simulink model "lab1"  (R2024b)
settings: Solver=VariableStepAuto  StartTime=0.0  StopTime=20  RelTol=1e-3
libraries: dspswit3 x2
settings Model: Creator=Ahmad  LastModifiedBy=Ahmad

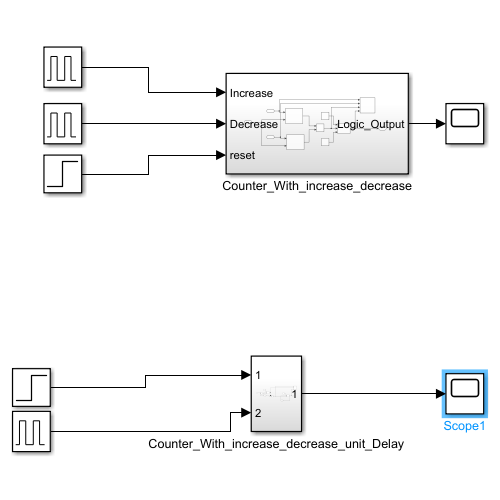
[thumbnail: Simulink's stored preview of the top-level diagram]
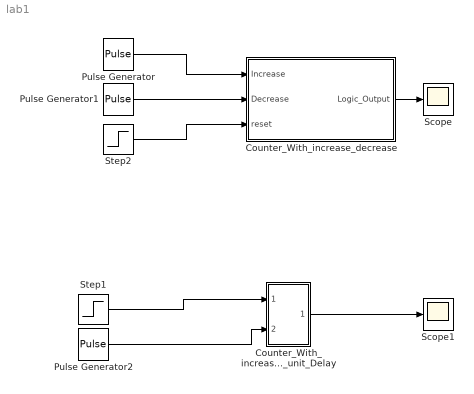
== system lab1 ==
  Counter_With_increase_decrease : Subsystem
  Counter_With_increase_decrease_unit_Delay : Subsystem
  Pulse Generator : DiscretePulseGenerator  PulseType=Time based  Period=1  PulseWidth=50
  Pulse Generator1 : DiscretePulseGenerator  PulseType=Time based  Period=6  PulseWidth=50
  Pulse Generator2 : DiscretePulseGenerator  PulseType=Time based  Period=6  PulseWidth=50
  Scope : Scope
  Scope1 : Scope
  Step1 : Step  SampleTime=1
  Step2 : Step  Time=8  SampleTime=0
  wires:
  Step1/1 -> Counter_With_increase_decrease_unit_Delay/1(In1)
  Pulse Generator/1 -> Counter_With_increase_decrease/1(Increase)
  Step2/1 -> Counter_With_increase_decrease/3(reset)
  Pulse Generator1/1 -> Counter_With_increase_decrease/2(Decrease)
  Counter_With_increase_decrease/1(Logic_Output) -> Scope/1
  Counter_With_increase_decrease_unit_Delay/1(Out1) -> Scope1/1
  Pulse Generator2/1 -> Counter_With_increase_decrease_unit_Delay/2(In2)

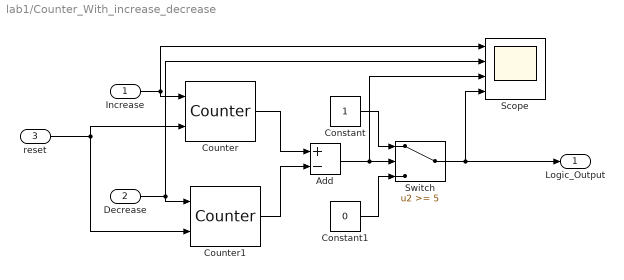
== system lab1/Counter_With_increase_decrease ==
  Increase : Inport
  Decrease : Inport  Port=2
  reset : Inport  Port=3
  Add : Sum  Inputs=+-
  Constant : Constant
  Constant1 : Constant  Value=0
  Counter : dspswit3/Counter  Direction=Up  CountEvent=Rising edge  CounterSize=User defined  MaxCount=255  InitialCount=0  Output=Count  HitValue=32  ResetInput=on  SamplesPerFrame=1  Ts=1  CntDtype=double  HitDtype=Logical
  Counter1 : dspswit3/Counter  Direction=Up  CountEvent=Rising edge  CounterSize=User defined  MaxCount=255  InitialCount=0  Output=Count  HitValue=32  ResetInput=on  SamplesPerFrame=1  Ts=1  CntDtype=double  HitDtype=Logical
  Scope : Scope  NumInputPorts=4
  Switch : Switch  Threshold=5  SaturateOnIntegerOverflow=off  InputSameDT=off
  Logic_Output : Outport
  wires:
  Decrease/1 -> Scope/2, Counter1/1
  Counter1/1 -> Add/2
  Add/1 -> Scope/3, Switch/2
  Increase/1 -> Scope/1, Counter/1
  reset/1 -> Counter1/2, Counter/2
  Counter/1 -> Add/1
  Constant1/1 -> Switch/3
  Constant/1 -> Switch/1
  Switch/1 -> Logic_Output/1, Scope/4

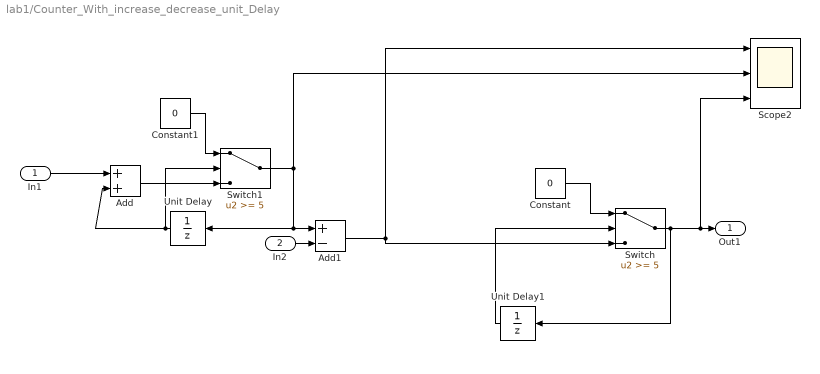
== system lab1/Counter_With_increase_decrease_unit_Delay ==
  In1 : Inport
  In2 : Inport  Port=2
  Add : Sum
  Add1 : Sum  Inputs=+-
  Constant : Constant  Value=0
  Constant1 : Constant  Value=0
  Scope2 : Scope  NumInputPorts=3
  Switch : Switch  Threshold=5  SaturateOnIntegerOverflow=off  InputSameDT=off
  Switch1 : Switch  Threshold=5  SaturateOnIntegerOverflow=off  InputSameDT=off
  Unit Delay : UnitDelay  SampleTime=-1  HasFrameUpgradeWarning=on
  Unit Delay1 : UnitDelay  SampleTime=-1  HasFrameUpgradeWarning=on
  Out1 : Outport
  wires:
  Unit Delay/1 -> Switch1/2, Add/2
  Add/1 -> Switch1/3
  Add1/1 -> Switch/3, Scope2/1
  Unit Delay1/1 -> Switch/2
  In1/1 -> Add/1
  Switch/1 -> Unit Delay1/1, Scope2/3, Out1/1
  Constant/1 -> Switch/1
  Switch1/1 -> Scope2/2, Unit Delay/1, Add1/1
  In2/1 -> Add1/2
  Constant1/1 -> Switch1/1
